simulink model "MotorXploer"  (R2024b)
settings: Solver=FixedStepAuto  StartTime=0.0  StopTime=inf  FixedStep=0.001  RelTol=1e-3
undefined symbols (not defined in the file or in its folder): Blocking, LF, Non
libraries: hdlsllib x5, amg_usbconverter_n_connect_lib x3
settings Model: Creator=beamk  LastModifiedBy=pboon

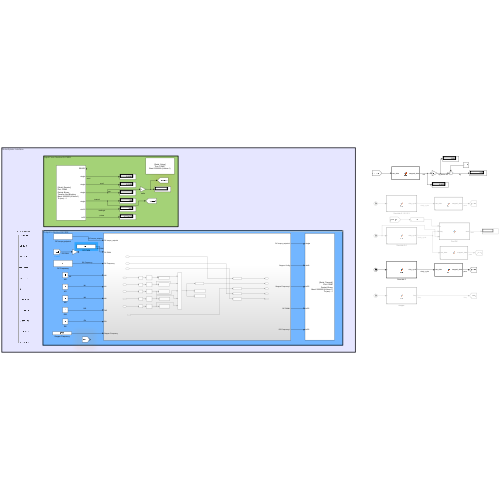
[thumbnail: Simulink's stored preview of the top-level diagram]
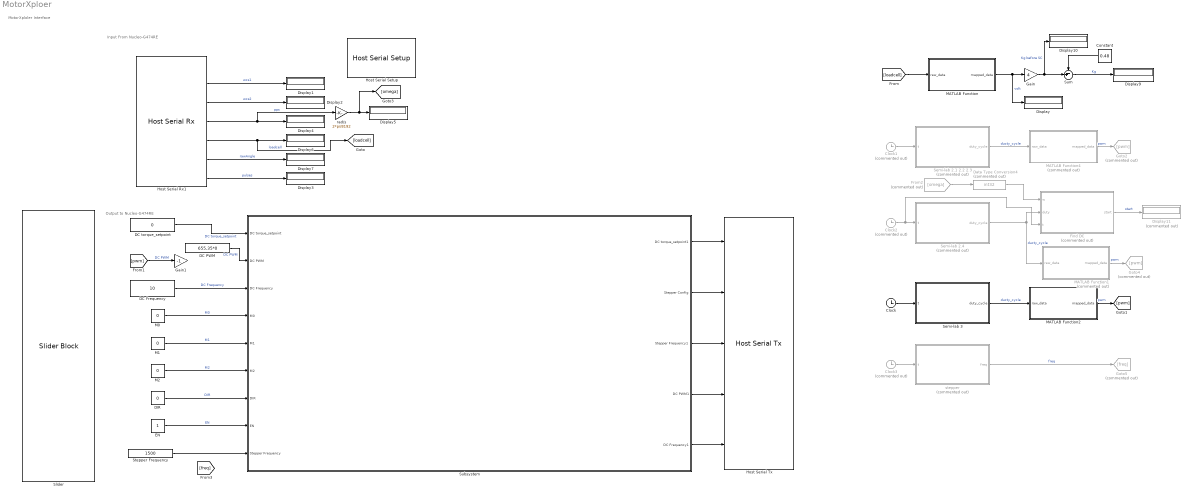
== system MotorXploer ==
  note: Output to Nucleo-G474RE
  note: Input From Nucleo-G474RE
  note: MotorXploler Interface
  Clock : Clock
  Clock1 : Clock  Commented=on
  Clock2 : Clock  Commented=on
  Clock3 : Clock  Commented=on
  Constant : Constant  Value=0.48
  DC Frequency : Constant  Value=10
  DC PWM : Constant  Value=655.35*0
  DC torque_setpoint : Constant  Value=0
  DIR : Constant  Value=0  OutDataTypeStr=uint8
  Data Type Conversion4 : DataTypeConversion  Commented=on  OutDataTypeStr=int32  SaturateOnIntegerOverflow=off  RndMeth=Floor
  Display{,1..7,9..10} (10 alike) : Display
      Display9 settings: Format=bank
  Display11 : Display  Commented=on
  EN : Constant  OutDataTypeStr=uint8
  Find DC : MATLAB Function  Commented=on  TreatAsAtomicUnit=on
  From2 : From  Commented=on  GotoTag=omega
  Gain : Gain  Gain=4
  Gain1 : Gain  Gain=-1
  Goto2 : Goto  Commented=on  GotoTag=pwm
  Goto4 : Goto  Commented=on  GotoTag=pwm
  Goto5 : Goto  Commented=on  GotoTag=freq
  Host Serial Rx1 : amg_usbconverter_n_connect_lib/Host Serial Rx  conf=rx  port=<auto>  baudrate=2000000  databits=8  parity=None  stopbit=1  flowcontrol=None  transfer=Non-Blocking  timeout=5  packetmode=Binary  enableinitialvalues=off  initialvalues=[]  binheader='45'  binterminator='A'  porttype_double=0  porttype_single=4  porttype_int8=0  porttype_uint8=0  porttype_int16=0  porttype_uint16=1  porttype_int32=1  porttype_uint32=0  asciiformat='%f,%f,%d,%d'  rx_asciiterminator="LF (0x0A - \"\\n\")"  tx_asciiterminator="CRLF (0x0D 0x0A - \"\\r\\n\")"  sampletime=-1  enablecustomportlabel=off  cinputportlabel=0  coutputportlabel=A  portpinstr=0  blockid=HostSerialRx1  inputporttype=[]  inputportwidth=[]  inputportlabel={}  outputporttype=[3 1 1 1 1 5 6]  outputportwidth=[1 1 1 1 1 1 1]  outputportlabel={'READY','single','single','single','single','uint16','int32'}  compat=0  optionstring=[]  autoport='COM5'
  Host Serial Setup : amg_usbconverter_n_connect_lib/Host Serial Setup  conf=setup  port=<auto>  baudrate=2000000  databits=8  parity=None  stopbit=1  flowcontrol=None  transfer=Blocking  timeout=2  packetmode=Binary  initialvalues=[]  binheader='7E 7E'  binterminator='03 03'  porttype_double=0  porttype_single=1  porttype_int8=0  porttype_uint8=0  porttype_int16=0  porttype_uint16=0  porttype_int32=0  porttype_uint32=2  asciiformat='%d %u %x'  rx_asciiterminator="CRLF (0x0D 0x0A - \"\\r\\n\")"  tx_asciiterminator="CRLF (0x0D 0x0A - \"\\r\\n\")"  sampletime=-1  enablecustomportlabel=off  cinputportlabel=0  coutputportlabel=A  portpinstr=0  blockid=HostSerialSetup  inputporttype=[]  inputportwidth=[]  inputportlabel={}  outputporttype=[]  outputportwidth=[]  outputportlabel={}  compat=0  optionstring=[]  autoport='COM5'
  Host Serial Tx : amg_usbconverter_n_connect_lib/Host Serial Tx  conf=tx  port=<auto>  baudrate=2000000  databits=8  parity=None  stopbit=1  flowcontrol=None  transfer=Blocking  timeout=2  packetmode=Binary  initialvalues=[]  binheader='45'  binterminator='A'  porttype_double=0  porttype_single=1  porttype_int8=0  porttype_uint8=1  porttype_int16=0  porttype_uint16=0  porttype_int32=3  porttype_uint32=0  asciiformat='%d,%f'  rx_asciiterminator="CRLF (0x0D 0x0A - \"\\r\\n\")"  tx_asciiterminator="CRLF (0x0D 0x0A - \"\\r\\n\")"  sampletime=-1  enablecustomportlabel=off  cinputportlabel=0  coutputportlabel=A  portpinstr=0  blockid=HostSerialTx  inputporttype=[1 3 6 6 6]  inputportwidth=[1 1 1 1 1]  inputportlabel={'single','uint8','int32','int32','int32'}  outputporttype=[]  outputportwidth=[]  outputportlabel={}  compat=0  optionstring=[]  autoport='COM5'
      settings: SourceProductName=aMG USB Converter N
  M0 : Constant  Value=0  OutDataTypeStr=uint8
  M1 : Constant  Value=0  OutDataTypeStr=uint8
  M2 : Constant  Value=0  OutDataTypeStr=uint8
  MATLAB Function : MATLAB Function  TreatAsAtomicUnit=on
  MATLAB Function1 : MATLAB Function  Commented=on  TreatAsAtomicUnit=on
  MATLAB Function2 : MATLAB Function  TreatAsAtomicUnit=on
  MATLAB Function4 : MATLAB Function  Commented=on  TreatAsAtomicUnit=on
  Semi-lab 2.1 2.2 2.3 : MATLAB Function  Commented=on  TreatAsAtomicUnit=on
  Semi-lab 2.4 : MATLAB Function  Commented=on  TreatAsAtomicUnit=on
  Semi-lab 3 : MATLAB Function  TreatAsAtomicUnit=on
  Slider : SliderBlock  ScaleMin=-65535  ScaleMax=65535
  Stepper Frequency : Constant  Value=1500
  Subsystem : Subsystem
  Sum : Sum  Inputs=-+|
  rad/s : Gain  Gain=2*pi/8192
  stepper : MATLAB Function  Commented=on  TreatAsAtomicUnit=on
  wires:
  rad/s/1 -> [omega], Display5/1
  Host Serial Rx1/7 -> Display3/1  "pulses"
  Host Serial Rx1/2 -> Display1/1  "wcs1"
  Host Serial Rx1/4 -> Display4/1, rad/s/1  "pps"
  Host Serial Rx1/3 -> Display2/1  "wcs2"
  Host Serial Rx1/5 -> [loadcell], Display6/1  "loadcell"
  Host Serial Rx1/6 -> Display7/1  "rawAngle"
  DC torque_setpoint/1 -> Subsystem/1(DC torque_setpoint)  "DC torque_setpoint"
  DC Frequency/1 -> Subsystem/3(DC Frequency)  "DC Frequency"
  M0/1 -> Subsystem/4(M0)  "M0"
  M1/1 -> Subsystem/5(M1)  "M1"
  M2/1 -> Subsystem/6(M2)  "M2"
  DIR/1 -> Subsystem/7(DIR)  "DIR"
  EN/1 -> Subsystem/8(EN)  "EN"
  Subsystem/1(DC torque_setpoint1) -> Host Serial Tx/1
  Subsystem/2(Stepper Config) -> Host Serial Tx/2
  Subsystem/3(Stepper Frequency1) -> Host Serial Tx/3
  Subsystem/4(DC PWM1) -> Host Serial Tx/4
  Subsystem/5(DC Frequency1) -> Host Serial Tx/5
  Clock/1 -> Semi-lab 3/1(t)
  Data Type Conversion4/1 -> Find DC/1(w)
  Sum/1 -> Display9/1  "Kg"
  From2/1 -> Data Type Conversion4/1
  MATLAB Function2/1(mapped_data) -> [pwm]  "pwm"
  Semi-lab 2.1 2.2 2.3/1(duty_cycle) -> MATLAB Function4/1(raw_data)  "ducty_cycle"
  Semi-lab 2.4/1(duty_cycle) -> Find DC/2(duty), MATLAB Function1/1(raw_data)  "ducty_cycle"
  Clock1/1 -> Semi-lab 2.1 2.2 2.3/1(t)
  Semi-lab 3/1(duty_cycle) -> MATLAB Function2/1(raw_data)  "ducty_cycle"
  Constant/1 -> Sum/1
  Find DC/1(start) -> Display11/1  "start"
  MATLAB Function/1(mapped_data) -> Display/1, Gain/1  "volt"
  MATLAB Function1/1(mapped_data) -> Goto4/1  "pwm"
  MATLAB Function4/1(mapped_data) -> Goto2/1  "pwm"
  Clock2/1 -> Find DC/3(t), Semi-lab 2.4/1(t)
  Gain/1 -> Display10/1, Sum/2  "Kg before SC"
  [loadcell] -> MATLAB Function/1(raw_data)
  stepper/1(freq) -> Goto5/1  "freq"
  Clock3/1 -> stepper/1(t)
  Stepper Frequency/1 -> Subsystem/9(Stepper Frequency)
  [pwm] -> Gain1/1  "DC PWM"
  DC PWM/1 -> Subsystem/2(DC PWM)  "DC PWM"

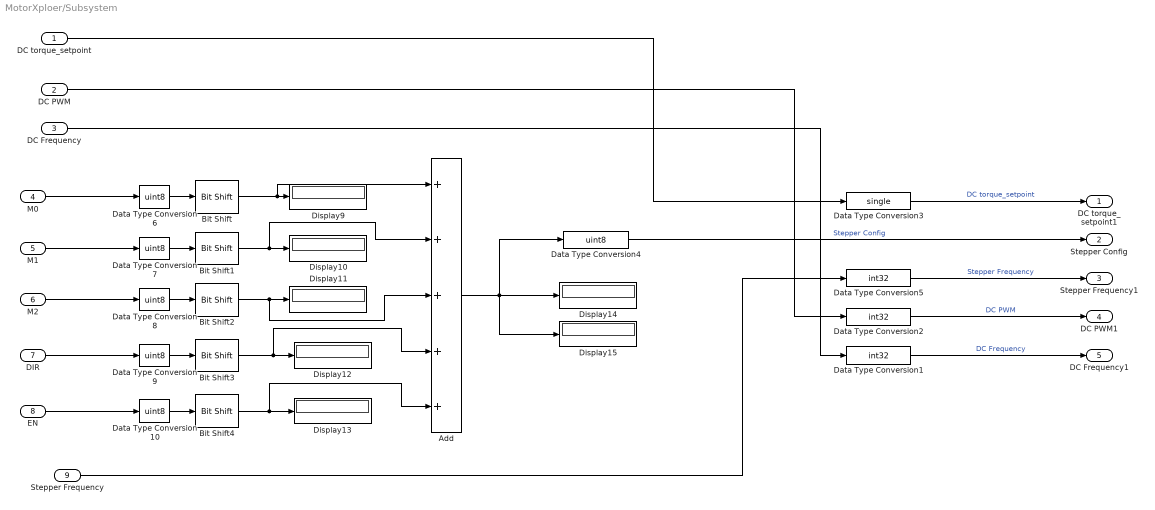
== system MotorXploer/Subsystem ==
  DC torque_setpoint : Inport
  DC PWM : Inport  Port=2
  DC Frequency : Inport  Port=3
  M0 : Inport  Port=4
  M1 : Inport  Port=5
  M2 : Inport  Port=6
  DIR : Inport  Port=7
  EN : Inport  Port=8
  Stepper Frequency : Inport  Port=9
  Add : Sum  Inputs=+++++
  Bit Shift : hdlsllib/Logic and Bit Operations/Bit Shift  mode=Shift Left Logical  N=4
  Bit Shift1 : hdlsllib/Logic and Bit Operations/Bit Shift  mode=Shift Left Logical  N=3
  Bit Shift2 : hdlsllib/Logic and Bit Operations/Bit Shift  mode=Shift Left Logical  N=2
  Bit Shift3 : hdlsllib/Logic and Bit Operations/Bit Shift  mode=Shift Left Logical  N=1
  Bit Shift4 : hdlsllib/Logic and Bit Operations/Bit Shift  mode=Shift Left Logical  N=0
  Data Type Conversion1 : DataTypeConversion  OutDataTypeStr=int32  SaturateOnIntegerOverflow=off  RndMeth=Floor
  Data Type Conversion{4,6..10} (6 alike) : DataTypeConversion  OutDataTypeStr=uint8  SaturateOnIntegerOverflow=off  RndMeth=Floor
  Data Type Conversion2 : DataTypeConversion  OutDataTypeStr=int32  SaturateOnIntegerOverflow=off  RndMeth=Floor
  Data Type Conversion3 : DataTypeConversion  OutDataTypeStr=single  SaturateOnIntegerOverflow=off  RndMeth=Floor
  Data Type Conversion5 : DataTypeConversion  OutDataTypeStr=int32  SaturateOnIntegerOverflow=off  RndMeth=Floor
  Display{9..15} (7 alike) : Display
      Display10 settings: Format=binary (Stored Integer)
      Display11 settings: Format=binary (Stored Integer)
      Display12 settings: Format=binary (Stored Integer)
      Display13 settings: Format=binary (Stored Integer)
      Display14 settings: Format=binary (Stored Integer)
      Display9 settings: Format=binary (Stored Integer)
  DC torque_setpoint1 : Outport
  Stepper Config : Outport  Port=2
  Stepper Frequency1 : Outport  Port=3
  DC PWM1 : Outport  Port=4
  DC Frequency1 : Outport  Port=5
  wires:
  Add/1 -> Data Type Conversion4/1, Display14/1, Display15/1
  M2/1 -> Data Type Conversion8/1
  DC Frequency/1 -> Data Type Conversion1/1
  Bit Shift3/1 -> Add/4, Display12/1
  Stepper Frequency/1 -> Data Type Conversion5/1
  Bit Shift2/1 -> Add/3, Display11/1
  Data Type Conversion7/1 -> Bit Shift1/1
  Data Type Conversion4/1 -> Stepper Config/1  "Stepper Config"
  Bit Shift/1 -> Add/1, Display9/1
  Data Type Conversion6/1 -> Bit Shift/1
  Data Type Conversion1/1 -> DC Frequency1/1  "DC Frequency"
  Data Type Conversion10/1 -> Bit Shift4/1
  Data Type Conversion2/1 -> DC PWM1/1  "DC PWM"
  Bit Shift4/1 -> Add/5, Display13/1
  Data Type Conversion8/1 -> Bit Shift2/1
  Data Type Conversion3/1 -> DC torque_setpoint1/1  "DC torque_setpoint"
  EN/1 -> Data Type Conversion10/1
  M0/1 -> Data Type Conversion6/1
  Bit Shift1/1 -> Add/2, Display10/1
  Data Type Conversion9/1 -> Bit Shift3/1
  DIR/1 -> Data Type Conversion9/1
  DC torque_setpoint/1 -> Data Type Conversion3/1
  DC PWM/1 -> Data Type Conversion2/1
  M1/1 -> Data Type Conversion7/1
  Data Type Conversion5/1 -> Stepper Frequency1/1  "Stepper Frequency"

== matlab function MotorXploer/MATLAB Function ==
  data: raw_data input; mapped_data output
function mapped_data = fcn(raw_data)

in_min = 0.0;
out_min = 0.0;
in_max = 4095.0;
out_max = 3.3;

mapped_data =  (double(raw_data) - in_min) * (out_max - out_min) / (in_max - in_min) + out_min;

== matlab function MotorXploer/MATLAB Function2 ==
  data: raw_data input; mapped_data output
function mapped_data = fcn(raw_data)

in_min = 0.0;
out_min = 0.0;
in_max = 100.0;
out_max = 65535.0;

mapped_data =  (double(raw_data) - in_min) * (out_max - out_min) / (in_max - in_min) + out_min;

== matlab function MotorXploer/Semi-lab 2.1 2.2 2.3 ==
  data: t input; duty_cycle output
function duty_cycle = fcn(t)

duty_cycle = 5*t;

== matlab function MotorXploer/MATLAB Function4 ==
  data: raw_data input; mapped_data output
function mapped_data = fcn(raw_data)

in_min = 0.0;
out_min = 0.0;
in_max = 100.0;
out_max = 65535.0;

mapped_data =  (double(raw_data) - in_min) * (out_max - out_min) / (in_max - in_min) + out_min;

== matlab function MotorXploer/Find DC ==
  data: w input; start output; duty input; t input
function start = fcn(w, duty, t)
persistent firstStartDuty firststopDuty

if isempty(firstStartDuty)
    firstStartDuty = NaN; 
end

if isempty(firststopDuty)
    firststopDuty = NaN; 
end

if w > 0.0 && isnan(firstStartDuty) && duty >= 1 && t <= 20
    firstStartDuty = duty;
    start = firstStartDuty;
elseif w == 0.0 && isnan(firststopDuty) && t > 20
    firststopDuty = duty;
    start = firststopDuty;
else
    start = 0.0;
end

== matlab function MotorXploer/Semi-lab 2.4 ==
  data: t input; duty_cycle output
function duty_cycle = fcn(t)
if t <= 20
    duty_cycle = 5 * t;
elseif t <= 40
    duty_cycle = 100 - (5 * (t - 20));
else
    duty_cycle = 0;
end

== matlab function MotorXploer/MATLAB Function1 ==
  data: raw_data input; mapped_data output
function mapped_data = fcn(raw_data)

in_min = 0.0;
out_min = 0.0;
in_max = 100.0;
out_max = 65535.0;

mapped_data =  (double(raw_data) - in_min) * (out_max - out_min) / (in_max - in_min) + out_min;

== matlab function MotorXploer/stepper ==
  data: t input; freq output
function freq = fcn(t)
freq = 10*t;

% 1/32 1/16 1000
% 1/8 500
% 1/4 250
% 1/2 100
% 1 10

== matlab function MotorXploer/Semi-lab 3 ==
  data: t input; duty_cycle output
function duty_cycle = fcn(t)
if t <= 20
    duty_cycle = 5 * t;
elseif t <= 40
    duty_cycle = 100 - (5 * (t - 20));
else
    duty_cycle = 0;
end

% function duty_cycle = fcn(t)
% duty_cycle_values = [50, 60, 70, 80, 90, 100, 90, 80, 70, 60, 50, 40, 30, 20, 10, 0, 10, 20, 30, 40, 50];
% 
% step_duration = 2.5; 
% 
% cycle_duration = numel(duty_cycle_values) * step_duration;
% 
% t_mod = mod(t, cycle_duration);
% 
% step_index = floor(t_mod / step_duration) + 1;
% 
% duty_cycle = duty_cycle_values(step_index);
